simulink model "quartercarmodel"  (R2024b)
settings: Solver=VariableStepAuto  StartTime=0.0  StopTime=10.0  RelTol=1e-3
values from neighbouring files (symbols this model uses):
  b = (sqrt((Tr_in(1) - Tr_out(1)).^2 + (Tr_in(2) - Tr_out(2)).^2))    [Max_Off_Axis_Rack_F.m]
  m = data{21,2}    [Max_Off_Axis_Rack_F.m]
undefined symbols (not defined in the file or in its folder): c
settings Model: Creator=rober  LastModifiedBy=rober

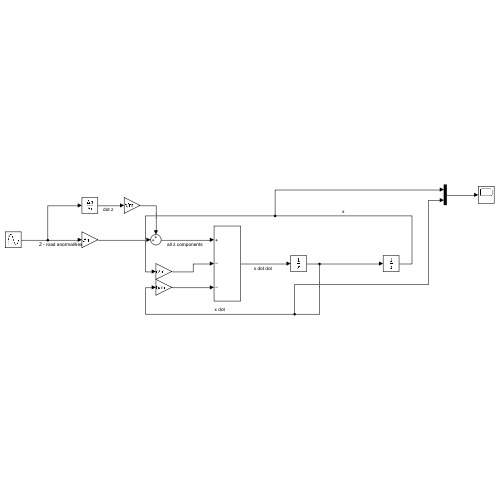
[thumbnail: Simulink's stored preview of the top-level diagram]
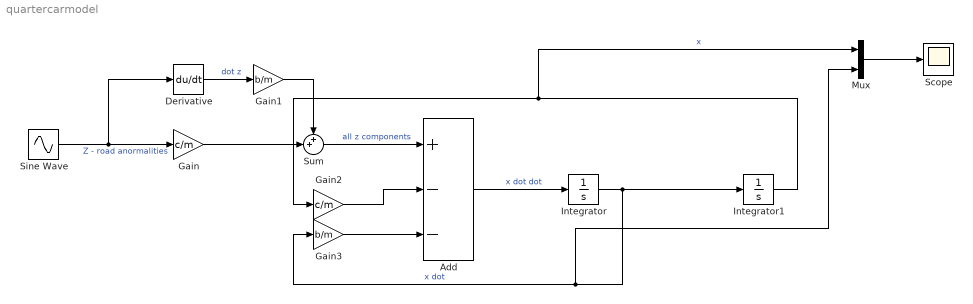
== system quartercarmodel ==
  Add : Sum  Inputs=+--
  Derivative : Derivative
  Gain : Gain  Gain=c/m
  Gain1 : Gain  Gain=b/m
  Gain2 : Gain  Gain=c/m
  Gain3 : Gain  Gain=b/m
  Integrator : Integrator
  Integrator1 : Integrator
  Mux : Mux  Inputs=2
  Scope : Scope
  Sine Wave : Sin  SampleTime=0
  Sum : Sum  Inputs=++|
  wires:
  Sine Wave/1 -> Derivative/1, Gain/1  "Z - road anormalities"
  Derivative/1 -> Gain1/1  "dot z"
  Gain1/1 -> Sum/1
  Gain/1 -> Sum/2
  Sum/1 -> Add/1  "all z components"
  Gain2/1 -> Add/2
  Gain3/1 -> Add/3
  Add/1 -> Integrator/1  "x dot dot"
  Integrator/1 -> Mux/2, Gain3/1, Integrator1/1  "x dot"
  Integrator1/1 -> Mux/1, Gain2/1  "x"
  Mux/1 -> Scope/1
